simulink model "rev_pow_ckt_new4"  (Simulink 10.0)
settings: Solver=ode23tb  StartTime=0.0  StopTime=10  RelTol=1e-3  EnableMultiTasking=on
libraries: powerlib x46, powerlib_extras x8, simulink x1
settings Model: Creator=Khan  LastModifiedBy=bhisma
settings DataIOCC: LimitDataPoints=on  SignalLoggingSaveFormat=ModelDataLogs
settings OptimizationCC: ExpressionDepthLimit=2147483647
settings DebuggingCC: SaveWithParameterizedLinksMsg=none  MultiTaskCondExecSysMsg=none  FcnCallInpInsideContextMsg=warning  StateNameClashWarn=warning
settings SFSimCC: SimParseCustomCode=off
settings GRTTargetCC: GeneratePreprocessorConditionals=Disable all
settings ConfigComp: CovExternalEMLEnable=off

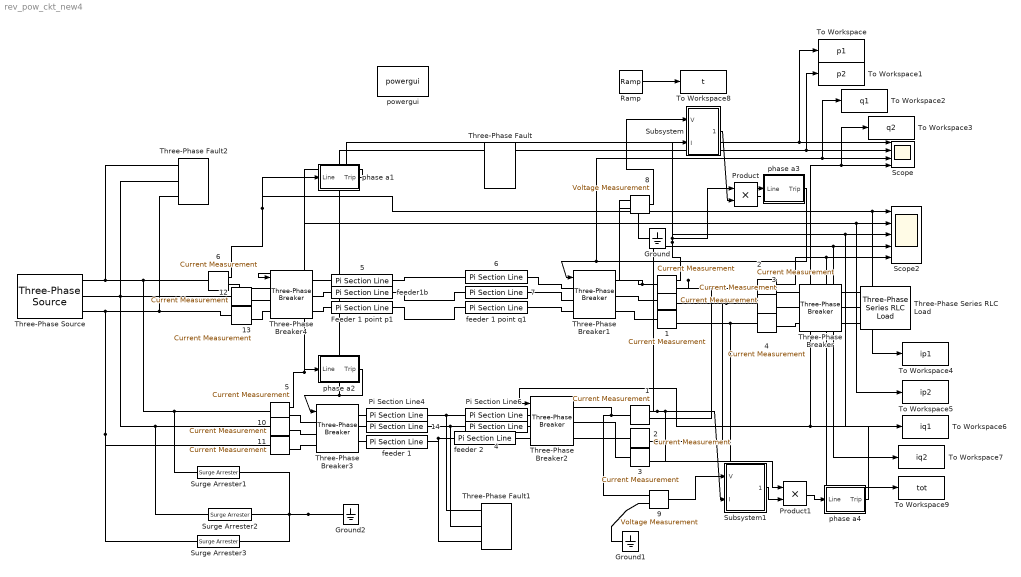
== system rev_pow_ckt_new4 ==
   {,1..3,10..13} (8 alike) : powerlib/Measurements/Current Measurement  SystemSampleTime=-1  PhasorSimulation=off  OutputType=Complex  PSBequivalent=0
      settings: SourceProductName=Simscape Electrical
    {,1..6} (7 alike) : powerlib/Measurements/Current Measurement  SystemSampleTime=-1  PhasorSimulation=off  OutputType=Complex  PSBequivalent=0
      settings: SourceProductName=Simscape Electrical
   {4..7,14} (5 alike) : powerlib/Elements/Pi Section Line  PhysicalDomain=powersysdomain  SubClassName=unknown  LeftPortType=p1  RightPortType=p1  LConnTagsString=__new0  RConnTagsString=__new0  Frequency=60  Resistance=0.2568  Inductance=2e-3  Capacitance=8.6e-9  Length=25  PiSections=1  Measurements=None
      settings: AttributesFormatString=\n  SourceProductName=Simscape Electrical  SourceProductBaseCode=PS
  " 8" : powerlib/Measurements/Voltage Measurement  SystemSampleTime=-1  PhasorSimulation=off  OutputType=Complex  PSBequivalent=0
      settings: SourceProductName=Simscape Electrical
  " 9" : powerlib/Measurements/Voltage Measurement  SystemSampleTime=-1  PhasorSimulation=off  OutputType=Complex  PSBequivalent=0
      settings: SourceProductName=Simscape Electrical
  Feeder 1 point p1 : powerlib/Elements/Pi Section Line  PhysicalDomain=powersysdomain  SubClassName=unknown  LeftPortType=p1  RightPortType=p1  LConnTagsString=__new0  RConnTagsString=__new0  Frequency=60  Resistance=0.2568  Inductance=2e-3  Capacitance=8.6e-9  Length=25  PiSections=1  Measurements=None
      settings: AttributesFormatString=\n  SourceProductName=Simscape Electrical  SourceProductBaseCode=PS
  Ground : powerlib/Elements/Ground  PhysicalDomain=powersysdomain  SubClassName=unknown  LeftPortType=p1  RightPortType=p1  LConnTagsString=a
      settings: SourceProductName=Simscape Electrical
  Ground1 : powerlib/Elements/Ground  PhysicalDomain=powersysdomain  SubClassName=unknown  LeftPortType=p1  RightPortType=p1  LConnTagsString=a
      settings: SourceProductName=Simscape Electrical
  Ground2 : powerlib/Elements/Ground  PhysicalDomain=powersysdomain  SubClassName=unknown  LeftPortType=p1  RightPortType=p1  LConnTagsString=a
      settings: SourceProductName=Simscape Electrical
  Pi Section Line4 : powerlib/Elements/Pi Section Line  PhysicalDomain=powersysdomain  SubClassName=unknown  LeftPortType=p1  RightPortType=p1  LConnTagsString=__new0  RConnTagsString=__new0  Frequency=60  Resistance=0.2568  Inductance=2e-3  Capacitance=8.6e-9  Length=25  PiSections=1  Measurements=None
      settings: AttributesFormatString=\n  SourceProductName=Simscape Electrical  SourceProductBaseCode=PS
  Pi Section Line6 : powerlib/Elements/Pi Section Line  PhysicalDomain=powersysdomain  SubClassName=unknown  LeftPortType=p1  RightPortType=p1  LConnTagsString=__new0  RConnTagsString=__new0  Frequency=60  Resistance=0.2568  Inductance=2e-3  Capacitance=8.6e-9  Length=25  PiSections=1  Measurements=None
      settings: AttributesFormatString=\n  SourceProductName=Simscape Electrical  SourceProductBaseCode=PS
  Product : Product  RndMeth=Zero
  Product1 : Product  RndMeth=Zero
  Ramp : simulink/Sources/Ramp  SystemSampleTime=-1  slope=1  start=0  X0=0
  Scope : Scope  NumInputPorts=4
  Scope2 : Scope  NumInputPorts=5
  Subsystem : Subsystem
  Subsystem1 : Subsystem
  Surge Arrester1 : powerlib/Elements/Surge Arrester  SystemSampleTime=-1  ProtectionVoltage=300e+03  Columns=2  ReferenceCurrent=500  Segment1=[.955 50]  Segment2=[1.0 25]  Segment3=[.9915 16.5]  Measurements=None  MoreParameters=off  BreakLoop=off
      settings: SourceProductName=Simscape Electrical  SourceProductBaseCode=PS
  Surge Arrester2 : powerlib/Elements/Surge Arrester  SystemSampleTime=-1  ProtectionVoltage=300e+03  Columns=2  ReferenceCurrent=500  Segment1=[.955 50]  Segment2=[1.0 25]  Segment3=[.9915 16.5]  Measurements=None  MoreParameters=off  BreakLoop=off
      settings: SourceProductName=Simscape Electrical  SourceProductBaseCode=PS
  Surge Arrester3 : powerlib/Elements/Surge Arrester  SystemSampleTime=-1  ProtectionVoltage=300e+03  Columns=2  ReferenceCurrent=500  Segment1=[.955 50]  Segment2=[1.0 25]  Segment3=[.9915 16.5]  Measurements=None  MoreParameters=off  BreakLoop=off
      settings: SourceProductName=Simscape Electrical  SourceProductBaseCode=PS
  Three-Phase Series RLC Load : powerlib/Elements/Three-Phase Series RLC Load  PhysicalDomain=powersysdomain  SubClassName=unknown  LeftPortType=p1  RightPortType=p1  LConnTagsString=A|B|C  Configuration=Y (grounded)  NominalVoltage=220e3  NominalFrequency=60  ActivePower=500e6  InductivePower=400e6  CapacitivePower=0  Measurements=None
      settings: SourceProductName=Simscape Electrical
  Three-Phase Breaker : powerlib/Elements/Three-Phase Breaker  SystemSampleTime=-1  InitialState=closed  SwitchA=on  SwitchB=on  SwitchC=on  SwitchTimes=100  External=off  BreakerResistance=0.001  SnubberResistance=1e6  SnubberCapacitance=inf  Measurements=None
      settings: SourceProductName=Simscape Electrical
  Three-Phase Breaker{1..4} (4 alike) : powerlib/Elements/Three-Phase Breaker  SystemSampleTime=-1  InitialState=closed  SwitchA=on  SwitchB=on  SwitchC=on  SwitchTimes=100  External=on  BreakerResistance=0.001  SnubberResistance=1e6  SnubberCapacitance=inf  Measurements=None
      settings: SourceProductName=Simscape Electrical
  Three-Phase Fault : powerlib/Elements/Three-Phase Fault  SystemSampleTime=-1  FaultA=on  FaultB=on  FaultC=on  FaultResistance=1  GroundFault=on  GroundResistance=0.001  External=off  SwitchStatus=1  SwitchTimes=4.998  InitialStates=[0 0 1]  SnubberResistance=1e6  SnubberCapacitance=inf  Measurements=None
      settings: SourceProductName=Simscape Electrical
  Three-Phase Fault1 : powerlib/Elements/Three-Phase Fault  SystemSampleTime=-1  FaultA=on  FaultB=on  FaultC=off  FaultResistance=1  GroundFault=on  GroundResistance=0.001  External=off  SwitchStatus=1  SwitchTimes=1.0022  InitialStates=[0 0 1]  SnubberResistance=1e6  SnubberCapacitance=inf  Measurements=None
      settings: SourceProductName=Simscape Electrical
  Three-Phase Fault2 : powerlib/Elements/Three-Phase Fault  SystemSampleTime=-1  FaultA=on  FaultB=on  FaultC=on  FaultResistance=1  GroundFault=on  GroundResistance=0.001  External=off  SwitchStatus=1  SwitchTimes=100  InitialStates=[0 0 1]  SnubberResistance=1e6  SnubberCapacitance=inf  Measurements=None
      settings: SourceProductName=Simscape Electrical
  Three-Phase Source : powerlib/Electrical Sources/Three-Phase Source  SystemSampleTime=-1  Voltage=220e3  PhaseAngle=0  Frequency=60  InternalConnection=Yg  SpecifyImpedance=off  Resistance=0.8929  Inductance=16.58e-3  ShortCircuitLevel=100e6  BaseVoltage=315e3  XRratio=7
      settings: SourceProductName=Simscape Electrical
  To Workspace : ToWorkspace  VariableName=p1  SampleTime=-1
  To Workspace1 : ToWorkspace  VariableName=p2  SampleTime=-1
  To Workspace2 : ToWorkspace  VariableName=q1  SampleTime=-1
  To Workspace3 : ToWorkspace  VariableName=q2  SampleTime=-1
  To Workspace4 : ToWorkspace  VariableName=ip1  SampleTime=-1
  To Workspace5 : ToWorkspace  VariableName=ip2  SampleTime=-1
  To Workspace6 : ToWorkspace  VariableName=iq1  SampleTime=-1
  To Workspace7 : ToWorkspace  VariableName=iq2  SampleTime=-1
  To Workspace8 : ToWorkspace  VariableName=t  SampleTime=-1
  To Workspace9 : ToWorkspace  VariableName=tot  SampleTime=-1
  feeder 1 : powerlib/Elements/Pi Section Line  PhysicalDomain=powersysdomain  SubClassName=unknown  LeftPortType=p1  RightPortType=p1  LConnTagsString=__new0  RConnTagsString=__new0  Frequency=60  Resistance=0.2568  Inductance=2e-3  Capacitance=8.6e-9  Length=25  PiSections=1  Measurements=None
      settings: AttributesFormatString=\n  SourceProductName=Simscape Electrical  SourceProductBaseCode=PS
  feeder 1 point q1 : powerlib/Elements/Pi Section Line  PhysicalDomain=powersysdomain  SubClassName=unknown  LeftPortType=p1  RightPortType=p1  LConnTagsString=__new0  RConnTagsString=__new0  Frequency=60  Resistance=0.2568  Inductance=2e-3  Capacitance=8.6e-9  Length=25  PiSections=1  Measurements=None
      settings: AttributesFormatString=\n  SourceProductName=Simscape Electrical  SourceProductBaseCode=PS
  feeder 2 : powerlib/Elements/Pi Section Line  PhysicalDomain=powersysdomain  SubClassName=unknown  LeftPortType=p1  RightPortType=p1  LConnTagsString=__new0  RConnTagsString=__new0  Frequency=60  Resistance=0.2568  Inductance=2e-3  Capacitance=8.6e-9  Length=25  PiSections=1  Measurements=None
      settings: AttributesFormatString=\n  SourceProductName=Simscape Electrical  SourceProductBaseCode=PS
  feeder1b : powerlib/Elements/Pi Section Line  PhysicalDomain=powersysdomain  SubClassName=unknown  LeftPortType=p1  RightPortType=p1  LConnTagsString=__new0  RConnTagsString=__new0  Frequency=60  Resistance=0.2568  Inductance=2e-3  Capacitance=8.6e-9  Length=25  PiSections=1  Measurements=None
      settings: AttributesFormatString=\n  SourceProductName=Simscape Electrical  SourceProductBaseCode=PS
  phase a1 : Subsystem
  phase a2 : Subsystem
  phase a3 : Subsystem
  phase a4 : Subsystem
  powergui : powerlib/powergui  Priority=1  SystemSampleTime=-1  SimulationMode=Continuous  SampleTime=50e-6  frequency=60  SPID=off  DisableSnubberDevices=off  DisableRonSwitches=off  DisableVfSwitches=off  SwTol=0  Interpol=off  frequencyindice=0  echomessages=off  HookPort=off  DisplayEquations=off  FunctionMessages=off  EnableUseOfTLC=off  x0status=blocks  RestoreLinks=warning  ResistiveCurrentMeasurement=off  Ylog=off  Xlog=on  ShowGrid=off  save=off  variable=ZData  ZoomFFT=off  StartTime=0.0  cycles=1  DisplayStyle=1  FreqAxis=off  MaxFrequency=1000  frequencyindicesteady=1  display=off  methode=off
      settings: SourceProductName=Simscape Electrical
  wires:
  " 8"/1 -> Subsystem/1(V)
  "  "/1 -> Subsystem/2(I), Product/1, Scope2/3, To Workspace6/1
  " 9"/1 -> Subsystem1/1(V)
  "  1"/1 -> Product1/1, Subsystem1/2(I), Scope2/4, To Workspace7/1
  Product/1 -> phase a3/1(Line)
  "  5"/1 -> phase a2/1(Line), Scope2/2, To Workspace5/1
  phase a2/1(Trip) -> Three-Phase Breaker3/1, To Workspace1/1, Scope/2
  "  6"/1 -> phase a1/1(Line), Scope2/1, To Workspace4/1
  phase a1/1(Trip) -> Three-Phase Breaker4/1, Scope/1, To Workspace/1
  Subsystem/1(Output) -> Product/2
  phase a3/1(Trip) -> Three-Phase Breaker1/1, Scope/3, To Workspace2/1
  Subsystem1/1(Output) -> Product1/2
  Product1/1 -> phase a4/1(Line)
  phase a4/1(Trip) -> Three-Phase Breaker2/1, Scope/4, To Workspace3/1
  "  2"/1 -> Scope2/5, To Workspace9/1
  Ramp/1 -> To Workspace8/1
  connections:
  "  2"/LConn1 -- "  1"/RConn1 -- "  "/RConn1
  "  3"/LConn1 -- " 2"/RConn1 -- " "/RConn1
  " 1"/RConn1 -- " 3"/RConn1 -- "  4"/LConn1
  " 6"/LConn1 -- " 5"/RConn1
  " 7"/LConn1 -- feeder1b/RConn1
  feeder 1 point q1/LConn1 -- Feeder 1 point p1/RConn1
  " 8"/LConn2 -- Ground/LConn1
  " 9"/LConn1 -- "  1"/LConn1 -- Three-Phase Breaker2/RConn1
  " 9"/LConn2 -- Ground1/LConn1
  Three-Phase Breaker/RConn1 -- Three-Phase Series RLC Load/LConn1
  Three-Phase Series RLC Load/LConn2 -- Three-Phase Breaker/RConn2
  Three-Phase Breaker/RConn3 -- Three-Phase Series RLC Load/LConn3
  "  2"/RConn1 -- Three-Phase Breaker/LConn1
  "  3"/RConn1 -- Three-Phase Breaker/LConn2
  "  4"/RConn1 -- Three-Phase Breaker/LConn3
  Three-Phase Breaker1/LConn1 -- " 6"/RConn1
  " 7"/RConn1 -- Three-Phase Breaker1/LConn2
  Three-Phase Breaker1/LConn3 -- feeder 1 point q1/RConn1
  "  "/LConn1 -- Three-Phase Breaker1/RConn1 -- " 8"/LConn1
  " "/LConn1 -- Three-Phase Breaker1/RConn2
  " 1"/LConn1 -- Three-Phase Breaker1/RConn3
  Three-Phase Breaker2/LConn1 -- Pi Section Line6/RConn1
  " 4"/RConn1 -- Three-Phase Breaker2/LConn2
  Three-Phase Breaker2/LConn3 -- feeder 2/RConn1
  Three-Phase Breaker2/RConn2 -- " 2"/LConn1
  Three-Phase Breaker2/RConn3 -- " 3"/LConn1
  "  5"/RConn1 -- Three-Phase Breaker3/LConn1
  " 10"/RConn1 -- Three-Phase Breaker3/LConn2
  " 11"/RConn1 -- Three-Phase Breaker3/LConn3
  " 12"/RConn1 -- Three-Phase Breaker4/LConn2
  " 13"/RConn1 -- Three-Phase Breaker4/LConn3
  "  6"/RConn1 -- Three-Phase Breaker4/LConn1
  Three-Phase Breaker4/RConn1 -- " 5"/LConn1
  Three-Phase Breaker4/RConn2 -- feeder1b/LConn1
  Three-Phase Breaker4/RConn3 -- Feeder 1 point p1/LConn1
  "  5"/LConn1 -- Surge Arrester1/LConn1 -- "  6"/LConn1 -- Three-Phase Source/RConn1 -- Three-Phase Fault2/LConn1
  Surge Arrester2/LConn1 -- " 12"/LConn1 -- Three-Phase Source/RConn2 -- Three-Phase Fault2/LConn2 -- " 10"/LConn1
  " 13"/LConn1 -- Surge Arrester3/LConn1 -- " 11"/LConn1 -- Three-Phase Source/RConn3 -- Three-Phase Fault2/LConn3
  Surge Arrester3/RConn1 -- Surge Arrester1/RConn1 -- Ground2/LConn1 -- Surge Arrester2/RConn1
  Pi Section Line4/LConn1 -- Three-Phase Breaker3/RConn1
  " 14"/LConn1 -- Three-Phase Breaker3/RConn2
  feeder 1/LConn1 -- Three-Phase Breaker3/RConn3
  Pi Section Line4/RConn1 -- Pi Section Line6/LConn1 -- Three-Phase Fault1/LConn1
  " 14"/RConn1 -- " 4"/LConn1 -- Three-Phase Fault1/LConn2
  feeder 1/RConn1 -- feeder 2/LConn1 -- Three-Phase Fault1/LConn3

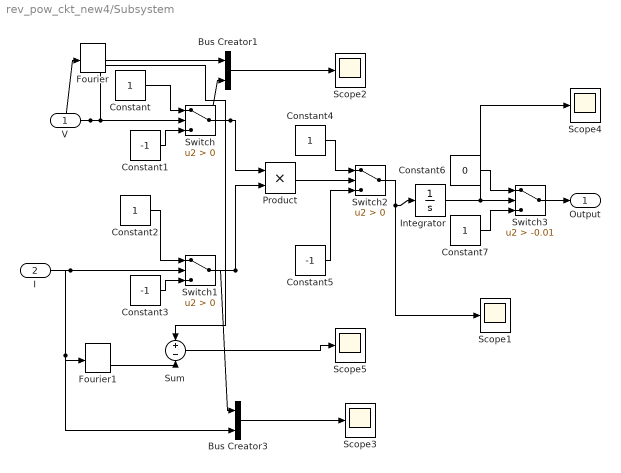
== system rev_pow_ckt_new4/Subsystem ==
  V : Inport
  I : Inport  Port=2
  Bus Creator1 : BusCreator  Inputs=2
  Bus Creator3 : BusCreator  Inputs=2
  Constant{,2,4,7} (4 alike) : Constant
  Constant1 : Constant  Value=-1
  Constant3 : Constant  Value=-1
  Constant5 : Constant  Value=-1
  Constant6 : Constant  Value=0
  Fourier : powerlib_extras/Measurements/Fourier  SystemSampleTime=-1  f1=60  n=1
      settings: SourceProductName=Simscape Electrical  SourceProductBaseCode=PS
  Fourier1 : powerlib_extras/Measurements/Fourier  SystemSampleTime=-1  f1=60  n=1
      settings: SourceProductName=Simscape Electrical  SourceProductBaseCode=PS
  Integrator : Integrator  LimitOutput=on  UpperSaturationLimit=0
  Product : Product  RndMeth=Zero
  Scope{1..5} (5 alike) : Scope
  Sum : Sum  Inputs=+-
  Switch : Switch  Criteria=u2 > Threshold
  Switch1 : Switch  Criteria=u2 > Threshold
  Switch2 : Switch  Criteria=u2 > Threshold
  Switch3 : Switch  Criteria=u2 > Threshold  Threshold=-0.01
  Output : Outport
  wires:
  Switch3/1 -> Output/1
  Constant7/1 -> Switch3/3
  Constant6/1 -> Switch3/1
  Integrator/1 -> Switch3/2, Scope4/1
  Bus Creator3/1 -> Scope3/1
  Bus Creator1/1 -> Scope2/1
  Switch2/1 -> Scope1/1, Integrator/1
  Constant5/1 -> Switch2/3
  Constant4/1 -> Switch2/1
  Product/1 -> Switch2/2
  Switch1/1 -> Bus Creator3/1, Product/2
  Switch/1 -> Bus Creator1/2, Product/1
  Constant3/1 -> Switch1/3
  Constant2/1 -> Switch1/1
  I/1 -> Bus Creator3/2, Fourier1/1, Switch1/2
  Constant1/1 -> Switch/3
  Constant/1 -> Switch/1
  V/1 -> Switch/2, Bus Creator1/1, Fourier/1
  Fourier/2 -> Sum/1
  Fourier1/2 -> Sum/2
  Sum/1 -> Scope5/1

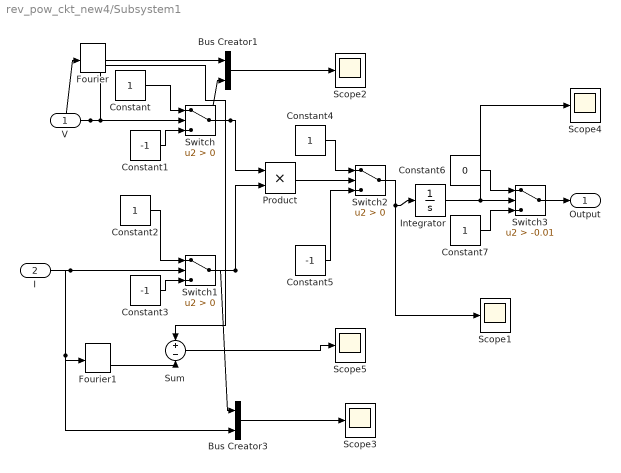
== system rev_pow_ckt_new4/Subsystem1 ==
  V : Inport
  I : Inport  Port=2
  Bus Creator1 : BusCreator  Inputs=2
  Bus Creator3 : BusCreator  Inputs=2
  Constant{,2,4,7} (4 alike) : Constant
  Constant1 : Constant  Value=-1
  Constant3 : Constant  Value=-1
  Constant5 : Constant  Value=-1
  Constant6 : Constant  Value=0
  Fourier : powerlib_extras/Measurements/Fourier  SystemSampleTime=-1  f1=60  n=1
      settings: SourceProductName=Simscape Electrical  SourceProductBaseCode=PS
  Fourier1 : powerlib_extras/Measurements/Fourier  SystemSampleTime=-1  f1=60  n=1
      settings: SourceProductName=Simscape Electrical  SourceProductBaseCode=PS
  Integrator : Integrator  LimitOutput=on  UpperSaturationLimit=0
  Product : Product  RndMeth=Zero
  Scope{1..5} (5 alike) : Scope
  Sum : Sum  Inputs=+-
  Switch : Switch  Criteria=u2 > Threshold
  Switch1 : Switch  Criteria=u2 > Threshold
  Switch2 : Switch  Criteria=u2 > Threshold
  Switch3 : Switch  Criteria=u2 > Threshold  Threshold=-0.01
  Output : Outport
  wires:
  Sum/1 -> Scope5/1
  Fourier1/2 -> Sum/2
  Fourier/2 -> Sum/1
  V/1 -> Fourier/1, Bus Creator1/1, Switch/2
  Constant/1 -> Switch/1
  Constant1/1 -> Switch/3
  I/1 -> Switch1/2, Fourier1/1, Bus Creator3/2
  Constant2/1 -> Switch1/1
  Constant3/1 -> Switch1/3
  Switch/1 -> Bus Creator1/2, Product/1
  Switch1/1 -> Bus Creator3/1, Product/2
  Product/1 -> Switch2/2
  Constant4/1 -> Switch2/1
  Constant5/1 -> Switch2/3
  Switch2/1 -> Integrator/1, Scope1/1
  Bus Creator1/1 -> Scope2/1
  Bus Creator3/1 -> Scope3/1
  Integrator/1 -> Scope4/1, Switch3/2
  Constant6/1 -> Switch3/1
  Constant7/1 -> Switch3/3
  Switch3/1 -> Output/1

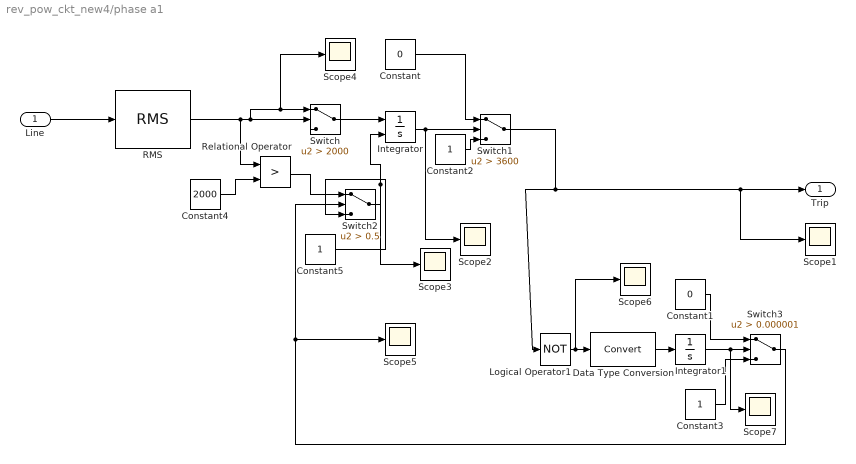
== system rev_pow_ckt_new4/phase a1 ==
  Line : Inport
  Constant : Constant  Value=0
  Constant1 : Constant  Value=0
  Constant2 : Constant
  Constant3 : Constant
  Constant4 : Constant  Value=2000
  Constant5 : Constant
  Data Type Conversion : DataTypeConversion
  Integrator : Integrator  ExternalReset=falling
  Integrator1 : Integrator
  Logical Operator1 : Logic  Operator=NOT  AllPortsSameDT=off  OutDataTypeStr=boolean
  RMS : powerlib_extras/Measurements/RMS  SystemSampleTime=-1  f1=60
      settings: SourceProductName=Simscape Electrical  SourceProductBaseCode=PS
  Relational Operator : RelationalOperator  Operator=>  OutDataTypeStr=boolean  RndMeth=Nearest
  Scope{1..7} (7 alike) : Scope
  Switch : Switch  Criteria=u2 > Threshold  Threshold=2000
  Switch1 : Switch  Criteria=u2 > Threshold  Threshold=3600  ZeroCross=off
  Switch2 : Switch  Criteria=u2 > Threshold  Threshold=0.5
  Switch3 : Switch  Criteria=u2 > Threshold  Threshold=0.000001
  Trip : Outport
  wires:
  Constant5/1 -> Switch2/3
  Switch2/1 -> Scope3/1, Integrator/2
  Relational Operator/1 -> Switch2/1
  Constant4/1 -> Relational Operator/2
  Constant3/1 -> Switch3/3
  Line/1 -> RMS/1
  Constant/1 -> Switch1/1
  Switch1/1 -> Logical Operator1/1, Trip/1, Scope1/1
  Integrator/1 -> Scope2/1, Switch1/2
  RMS/1 -> Relational Operator/1, Switch/2, Scope4/1, Switch/1
  Switch/1 -> Integrator/1
  Constant2/1 -> Switch1/3
  Logical Operator1/1 -> Scope6/1, Data Type Conversion/1
  Data Type Conversion/1 -> Integrator1/1
  Integrator1/1 -> Scope7/1, Switch3/2
  Constant1/1 -> Switch3/1
  Switch3/1 -> Switch2/2, Scope5/1

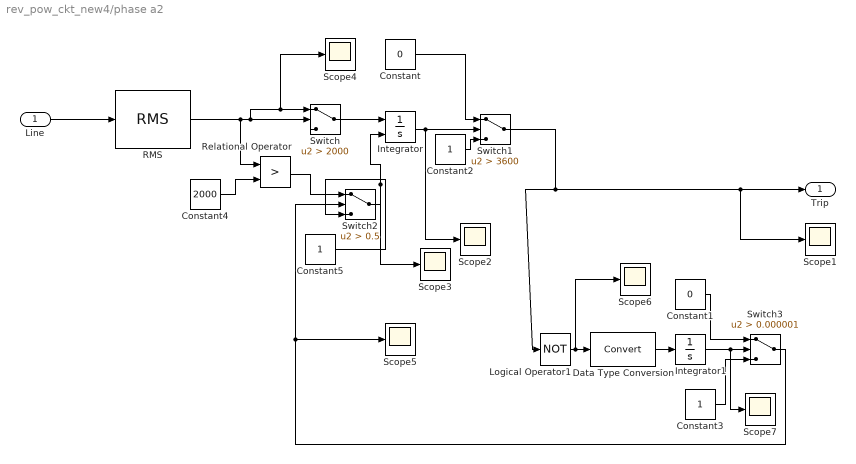
== system rev_pow_ckt_new4/phase a2 ==
  Line : Inport
  Constant : Constant  Value=0
  Constant1 : Constant  Value=0
  Constant2 : Constant
  Constant3 : Constant
  Constant4 : Constant  Value=2000
  Constant5 : Constant
  Data Type Conversion : DataTypeConversion
  Integrator : Integrator  ExternalReset=falling
  Integrator1 : Integrator
  Logical Operator1 : Logic  Operator=NOT  AllPortsSameDT=off  OutDataTypeStr=boolean
  RMS : powerlib_extras/Measurements/RMS  SystemSampleTime=-1  f1=60
      settings: SourceProductName=Simscape Electrical  SourceProductBaseCode=PS
  Relational Operator : RelationalOperator  Operator=>  OutDataTypeStr=boolean  RndMeth=Nearest
  Scope{1..7} (7 alike) : Scope
  Switch : Switch  Criteria=u2 > Threshold  Threshold=2000
  Switch1 : Switch  Criteria=u2 > Threshold  Threshold=3600  ZeroCross=off
  Switch2 : Switch  Criteria=u2 > Threshold  Threshold=0.5
  Switch3 : Switch  Criteria=u2 > Threshold  Threshold=0.000001
  Trip : Outport
  wires:
  Switch3/1 -> Scope5/1, Switch2/2
  Constant1/1 -> Switch3/1
  Integrator1/1 -> Switch3/2, Scope7/1
  Data Type Conversion/1 -> Integrator1/1
  Logical Operator1/1 -> Data Type Conversion/1, Scope6/1
  Constant2/1 -> Switch1/3
  Switch/1 -> Integrator/1
  RMS/1 -> Scope4/1, Switch/1, Switch/2, Relational Operator/1
  Integrator/1 -> Switch1/2, Scope2/1
  Switch1/1 -> Scope1/1, Trip/1, Logical Operator1/1
  Constant/1 -> Switch1/1
  Line/1 -> RMS/1
  Constant3/1 -> Switch3/3
  Constant4/1 -> Relational Operator/2
  Relational Operator/1 -> Switch2/1
  Switch2/1 -> Integrator/2, Scope3/1
  Constant5/1 -> Switch2/3

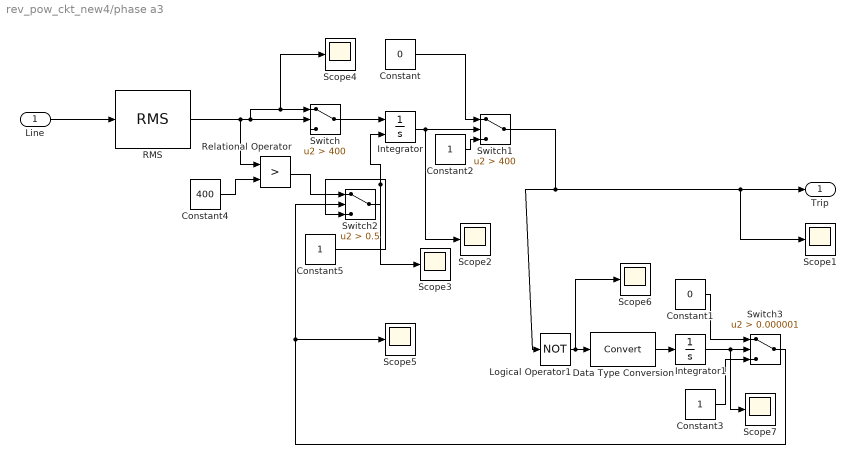
== system rev_pow_ckt_new4/phase a3 ==
  Line : Inport
  Constant : Constant  Value=0
  Constant1 : Constant  Value=0
  Constant2 : Constant
  Constant3 : Constant
  Constant4 : Constant  Value=400
  Constant5 : Constant
  Data Type Conversion : DataTypeConversion
  Integrator : Integrator  ExternalReset=falling
  Integrator1 : Integrator
  Logical Operator1 : Logic  Operator=NOT  AllPortsSameDT=off  OutDataTypeStr=boolean
  RMS : powerlib_extras/Measurements/RMS  SystemSampleTime=-1  f1=60
      settings: SourceProductName=Simscape Electrical  SourceProductBaseCode=PS
  Relational Operator : RelationalOperator  Operator=>  OutDataTypeStr=boolean  RndMeth=Nearest
  Scope{1..7} (7 alike) : Scope
  Switch : Switch  Criteria=u2 > Threshold  Threshold=400
  Switch1 : Switch  Criteria=u2 > Threshold  Threshold=400  ZeroCross=off
  Switch2 : Switch  Criteria=u2 > Threshold  Threshold=0.5
  Switch3 : Switch  Criteria=u2 > Threshold  Threshold=0.000001
  Trip : Outport
  wires:
  Switch3/1 -> Scope5/1, Switch2/2
  Constant1/1 -> Switch3/1
  Integrator1/1 -> Switch3/2, Scope7/1
  Data Type Conversion/1 -> Integrator1/1
  Logical Operator1/1 -> Data Type Conversion/1, Scope6/1
  Constant2/1 -> Switch1/3
  Switch/1 -> Integrator/1
  RMS/1 -> Scope4/1, Switch/1, Switch/2, Relational Operator/1
  Integrator/1 -> Switch1/2, Scope2/1
  Switch1/1 -> Scope1/1, Trip/1, Logical Operator1/1
  Constant/1 -> Switch1/1
  Line/1 -> RMS/1
  Constant3/1 -> Switch3/3
  Constant4/1 -> Relational Operator/2
  Relational Operator/1 -> Switch2/1
  Switch2/1 -> Integrator/2, Scope3/1
  Constant5/1 -> Switch2/3

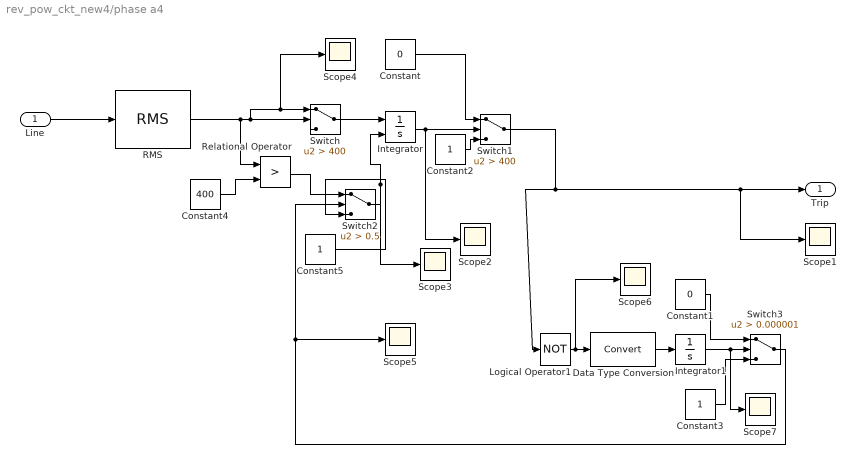
== system rev_pow_ckt_new4/phase a4 ==
  Line : Inport
  Constant : Constant  Value=0
  Constant1 : Constant  Value=0
  Constant2 : Constant
  Constant3 : Constant
  Constant4 : Constant  Value=400
  Constant5 : Constant
  Data Type Conversion : DataTypeConversion
  Integrator : Integrator  ExternalReset=falling
  Integrator1 : Integrator
  Logical Operator1 : Logic  Operator=NOT  AllPortsSameDT=off  OutDataTypeStr=boolean
  RMS : powerlib_extras/Measurements/RMS  SystemSampleTime=-1  f1=60
      settings: SourceProductName=Simscape Electrical  SourceProductBaseCode=PS
  Relational Operator : RelationalOperator  Operator=>  OutDataTypeStr=boolean  RndMeth=Nearest
  Scope{1..7} (7 alike) : Scope
  Switch : Switch  Criteria=u2 > Threshold  Threshold=400
  Switch1 : Switch  Criteria=u2 > Threshold  Threshold=400  ZeroCross=off
  Switch2 : Switch  Criteria=u2 > Threshold  Threshold=0.5
  Switch3 : Switch  Criteria=u2 > Threshold  Threshold=0.000001
  Trip : Outport
  wires:
  Constant5/1 -> Switch2/3
  Switch2/1 -> Scope3/1, Integrator/2
  Relational Operator/1 -> Switch2/1
  Constant4/1 -> Relational Operator/2
  Constant3/1 -> Switch3/3
  Line/1 -> RMS/1
  Constant/1 -> Switch1/1
  Switch1/1 -> Logical Operator1/1, Trip/1, Scope1/1
  Integrator/1 -> Scope2/1, Switch1/2
  RMS/1 -> Relational Operator/1, Switch/2, Switch/1, Scope4/1
  Switch/1 -> Integrator/1
  Constant2/1 -> Switch1/3
  Logical Operator1/1 -> Scope6/1, Data Type Conversion/1
  Data Type Conversion/1 -> Integrator1/1
  Integrator1/1 -> Scope7/1, Switch3/2
  Constant1/1 -> Switch3/1
  Switch3/1 -> Switch2/2, Scope5/1
